simulink model "bilateral_control_not_wv"  (R2023a)
settings: Solver=VariableStepAuto  StartTime=0.0  StopTime=100  RelTol=1e-3
settings Model: Creator=UPM  LastModifiedBy=Josep

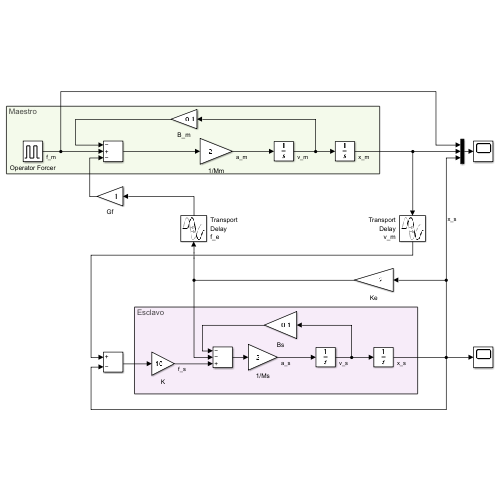
[thumbnail: Simulink's stored preview of the top-level diagram]
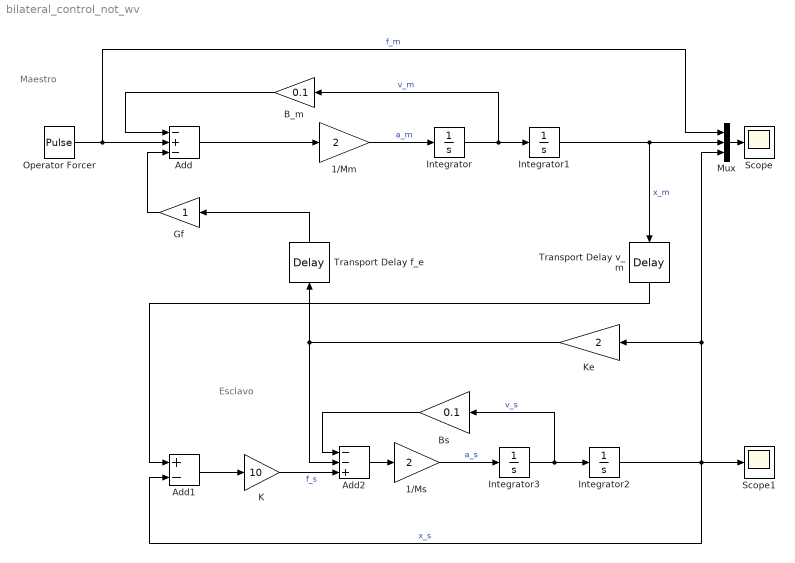
== system bilateral_control_not_wv ==
  note: Esclavo
  note: Maestro
  1/Mm : Gain  Gain=2
  1/Ms : Gain  Gain=2
  Add : Sum  Inputs=-+-
  Add1 : Sum  Inputs=+-
  Add2 : Sum  Inputs=--+
  B_m : Gain  Gain=0.1
  Bs : Gain  Gain=0.1
  Gf : Gain
  Integrator{,1..3} (4 alike) : Integrator
  K : Gain  Gain=10
  Ke : Gain  Gain=2
  Mux : Mux  Inputs=3
  Operator Forcer : DiscretePulseGenerator  PulseType=Time based  Amplitude=4  Period=40  PulseWidth=50
  Scope : Scope
  Scope1 : Scope
  Transport Delay f_e : TransportDelay  DelayTime=0.05
  Transport Delay v_m : TransportDelay  DelayTime=0.05
  wires:
  Integrator3/1 -> Integrator2/1, Bs/1  "v_s"
  1/Mm/1 -> Integrator/1  "a_m"
  Integrator2/1 -> Ke/1, Mux/3, Scope1/1, Add1/2  "x_s"
  1/Ms/1 -> Integrator3/1  "a_s"
  Add1/1 -> K/1
  K/1 -> Add2/3  "f_s"
  Add2/1 -> 1/Ms/1
  Bs/1 -> Add2/1
  Add/1 -> 1/Mm/1
  Ke/1 -> Transport Delay f_e/1, Add2/2
  Operator Forcer/1 -> Mux/1, Add/2  "f_m"
  B_m/1 -> Add/1
  Gf/1 -> Add/3
  Integrator1/1 -> Mux/2, Transport Delay v_m/1  "x_m"
  Mux/1 -> Scope/1
  Transport Delay f_e/1 -> Gf/1
  Transport Delay v_m/1 -> Add1/1
  Integrator/1 -> B_m/1, Integrator1/1  "v_m"
